simulink model "vlacik_model"  (Simulink 7.5)
settings: Solver=ode45  StartTime=0.0  StopTime=300  RelTol=1e-3
values from neighbouring files (symbols this model uses):
  K = place(Anew, Bnew, [roots(char);-5;-6])    [helikoptera.m]    (also in matlab_workspace.mat = [-0.0736632883088 0.867498250153 -0.0253045109983 7.04683660; priklad.m = acker(A,B,[-0.0400+0.0419*i, -0.0400-0.0419*i, -0.5, 0]))
  sys = ss(A,B,C,0)    [helikoptera.m]    (also in matlab_workspace.mat = ; priklad.m; vagon.m = ss(A,B,C,D))
  sysState = ss(A-B*K,B,C,0)    [priklad.m]
libraries: simulink x2
settings Model: Creator=michal  LastModifiedBy=michal

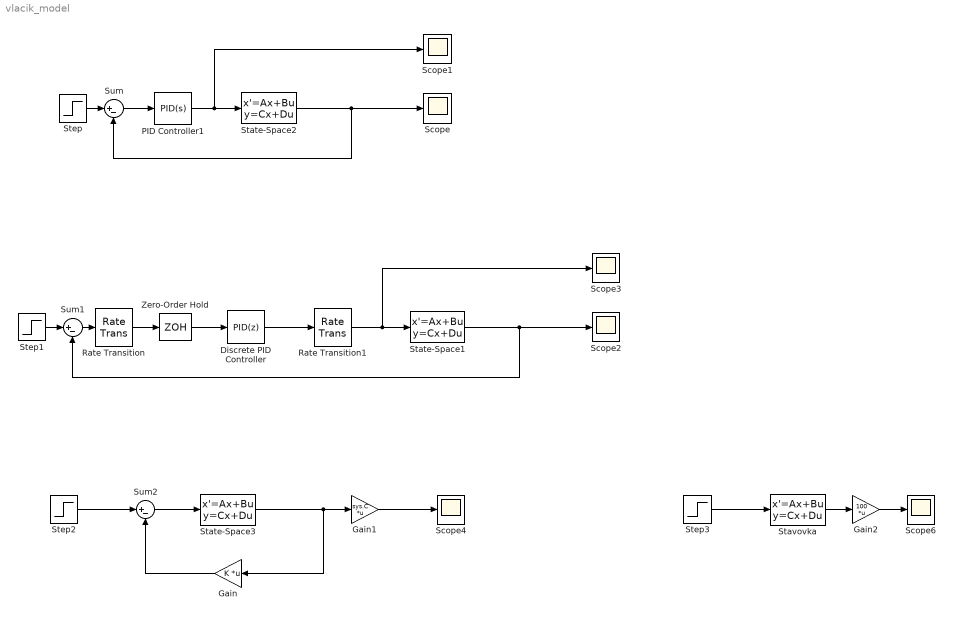
== system vlacik_model ==
  Discrete PID Controller : simulink/Continuous/PID Controller  DialogController=pidpack.PIDConfig.pidDDGCreate  DialogControllerArgs=DataTag0  SystemSampleTime=-1  Controller=PID  TimeDomain=Discrete-time  SampleTime=1  IntegratorMethod=Forward Euler  FilterMethod=Forward Euler  Form=Parallel  P=2000  I=100  D=0  N=100  InitialConditionSource=internal  InitialConditionForIntegrator=0  InitialConditionForFilter=0  ExternalReset=none  LimitOutput=on  UpperSaturationLimit=62000  LowerSaturationLimit=0  LinearizeAsGain=off  AntiWindupMode=none  Kb=1  TrackingMode=off  Kt=1  PParamMin=[]  PParamMax=[]  IParamMin=[]  IParamMax=[]  DParamMin=[]  DParamMax=[]  NParamMin=[]  NParamMax=[]  KbParamMin=[]  KbParamMax=[]  KtParamMin=[]  KtParamMax=[]  POutMin=[]  POutMax=[]  IOutMin=[]  IOutMax=[]  DOutMin=[]  DOutMax=[]  NOutMin=[]  NOutMax=[]  KbOutMin=[]  KbOutMax=[]  KtOutMin=[]  KtOutMax=[]  IntegratorOutMin=[]  IntegratorOutMax=[]  FilterOutMin=[]  FilterOutMax=[]  SumOutMin=[]  SumOutMax=[]  SumI1OutMin=[]  SumI1OutMax=[]  SumI2OutMin=[]  SumI2OutMax=[]  SumI3OutMin=[]  SumI3OutMax=[]  SumDOutMin=[]  SumDOutMax=[]  SaturationOutMin=[]  SaturationOutMax=[]  IntegratorContinuousStateAttributes=''  IntegratorStateMustResolveToSignalObject=off  IntegratorRTWStateStorageClass=Auto  FilterContinuousStateAttributes=''  FilterStateMustResolveToSignalObject=off  FilterRTWStateStorageClass=Auto
  Gain : Gain  Gain=K  Multiplication=Matrix(K*u)  ParameterDataType=fixdt(1, 16)  ParameterScaling=2^0  OutDataType=fixdt(1, 16)  OutScaling=2^0
  Gain1 : Gain  Gain=sys.C  Multiplication=Matrix(K*u)  ParameterDataType=fixdt(1, 16)  ParameterScaling=2^0  OutDataType=fixdt(1, 16)  OutScaling=2^0
  Gain2 : Gain  Gain=100  Multiplication=Matrix(K*u)  ParameterDataType=fixdt(1, 16)  ParameterScaling=2^0  OutDataType=fixdt(1, 16)  OutScaling=2^0
  PID Controller1 : simulink/Continuous/PID Controller  DialogController=pidpack.PIDConfig.pidDDGCreate  DialogControllerArgs=DataTag1  SystemSampleTime=-1  Controller=PID  TimeDomain=Continuous-time  SampleTime=1  IntegratorMethod=Forward Euler  FilterMethod=Forward Euler  Form=Parallel  P=2000  I=100  D=0  N=100  InitialConditionSource=internal  InitialConditionForIntegrator=0  InitialConditionForFilter=0  ExternalReset=none  LimitOutput=on  UpperSaturationLimit=62000  LowerSaturationLimit=0  LinearizeAsGain=off  AntiWindupMode=none  Kb=1  TrackingMode=off  Kt=1  PParamMin=[]  PParamMax=[]  IParamMin=[]  IParamMax=[]  DParamMin=[]  DParamMax=[]  NParamMin=[]  NParamMax=[]  KbParamMin=[]  KbParamMax=[]  KtParamMin=[]  KtParamMax=[]  POutMin=[]  POutMax=[]  IOutMin=[]  IOutMax=[]  DOutMin=[]  DOutMax=[]  NOutMin=[]  NOutMax=[]  KbOutMin=[]  KbOutMax=[]  KtOutMin=[]  KtOutMax=[]  IntegratorOutMin=[]  IntegratorOutMax=[]  FilterOutMin=[]  FilterOutMax=[]  SumOutMin=[]  SumOutMax=[]  SumI1OutMin=[]  SumI1OutMax=[]  SumI2OutMin=[]  SumI2OutMax=[]  SumI3OutMin=[]  SumI3OutMax=[]  SumDOutMin=[]  SumDOutMax=[]  SaturationOutMin=[]  SaturationOutMax=[]  IntegratorContinuousStateAttributes=''  IntegratorStateMustResolveToSignalObject=off  IntegratorRTWStateStorageClass=Auto  FilterContinuousStateAttributes=''  FilterStateMustResolveToSignalObject=off  FilterRTWStateStorageClass=Auto
  Rate Transition : RateTransition  OutPortSampleTime=1
  Rate Transition1 : RateTransition  OutPortSampleTime=1
  Scope{,1..4,6} (6 alike) : Scope
      Scope settings: TimeRange=300  YMin=14.9997  YMax=15
      Scope1 settings: YMin=-56  YMax=-37
      Scope2 settings: YMin=14.9997  YMax=15  SaveName=ScopeData2
      Scope3 settings: YMin=-56  YMax=-37  SaveName=ScopeData3
      Scope4 settings: YMin=0  YMax=8e-06  SaveName=ScopeData4
      Scope6 settings: YMin=0  YMax=8e-06  SaveName=ScopeData6
  State-Space1 : StateSpace  A=sys.a  B=sys.b  C=sys.c  D=sys.d
  State-Space2 : StateSpace  A=sys.a  B=sys.b  C=sys.c  D=sys.d
  State-Space3 : StateSpace  A=sys.a  B=sys.b  C=eye(4)  D=[0 0 0 0]'
  Stavovka : StateSpace  A=sysState.a  B=sysState.b  C=sysState.c  D=sysState.d
  Step : Step  Time=0  After=15  SampleTime=0
  Step1 : Step  Time=0  After=15  SampleTime=0
  Step2 : Step  Time=0  After=15  SampleTime=0
  Step3 : Step  Time=0  After=10  SampleTime=0
  Sum : Sum  Inputs=|+-  OutDataType=fixdt(1, 16)  OutScaling=2^0
  Sum1 : Sum  Inputs=|+-  OutDataType=fixdt(1, 16)  OutScaling=2^0
  Sum2 : Sum  Inputs=|+-  OutDataType=fixdt(1, 16)  OutScaling=2^0
  Zero-Order Hold : ZeroOrderHold
  wires:
  State-Space2/1 -> Scope/1, Sum/2
  Step/1 -> Sum/1
  Sum/1 -> PID Controller1/1
  PID Controller1/1 -> State-Space2/1, Scope1/1
  State-Space1/1 -> Scope2/1, Sum1/2
  Step1/1 -> Sum1/1
  Sum1/1 -> Rate Transition/1
  Rate Transition/1 -> Zero-Order Hold/1
  Discrete PID Controller/1 -> Rate Transition1/1
  Zero-Order Hold/1 -> Discrete PID Controller/1
  Rate Transition1/1 -> State-Space1/1, Scope3/1
  State-Space3/1 -> Gain/1, Gain1/1
  Sum2/1 -> State-Space3/1
  Gain/1 -> Sum2/2
  Gain1/1 -> Scope4/1
  Step2/1 -> Sum2/1
  Step3/1 -> Stavovka/1
  Stavovka/1 -> Gain2/1
  Gain2/1 -> Scope6/1
